simulink model "EvenOrOdd"  (R2021a)
settings: Solver=FixedStepDiscrete  StartTime=0.0  StopTime=10.0  RelTol=1e-3
settings Model: Creator=OmarMedhat  LastModifiedBy=OmarMedhat
settings OptimizationCC: DefaultParameterBehavior=Inlined  EnhancedBackFolding=on  PassReuseOutputArgsAs=Individual arguments  ZeroExternalMemoryAtStartup=off  ZeroInternalMemoryAtStartup=off  OptimizeBlockOrder=speed  DifferentSizesBufferReuse=on  OptimizationCustomize=off  EfficientTunableParamExpr=on
settings DebuggingCC: ParameterTunabilityLossMsg=error
settings SFSimCC: MATLABDynamicMemAlloc=off
settings RTWCC: SystemTargetFile=ert.tlc  GenCodeOnly=on  TemplateMakefile=ert_default_tmf  GenerateReport=on  IncludeHyperlinkInReport=on  LaunchReport=on  GenerateTraceInfo=on
settings CodeAppCC: ForceParamTrailComments=on  IgnoreCustomStorageClasses=off  OperatorAnnotations=on  SimulinkDataObjDesc=on  SFDataObjDesc=on  InsertBlockDesc=on
settings ERTTargetCC: TargetLangStandard=C99 (ISO)  GenerateSampleERTMain=on  InlinedParameterPlacement=NonHierarchical  ERTCustomFileTemplate=example_file_process.tlc

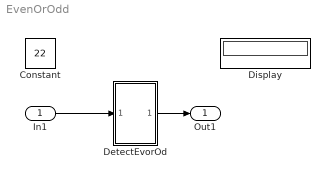
== system EvenOrOdd ==
  In1 : Inport
  Constant : Constant  Value=22
  DetectEvorOd : Subsystem  TreatAsAtomicUnit=on
      settings: RTWFcnNameOpts=Use subsystem name  RTWFileNameOpts=Use subsystem name
  Display : Display
  Out1 : Outport
  wires:
  In1/1 -> DetectEvorOd/1(In1)
  DetectEvorOd/1(Out1) -> Out1/1

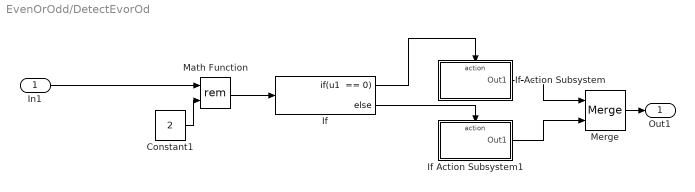
== system EvenOrOdd/DetectEvorOd ==
  In1 : Inport
  Constant1 : Constant  Value=2
  If : If  IfExpression="u1  == 0"
  If Action Subsystem : Subsystem  TreatAsAtomicUnit=on
  If Action Subsystem1 : Subsystem  TreatAsAtomicUnit=on
  Math Function : Math  Operator=rem  SaturateOnIntegerOverflow=on
  Merge : Merge
  Out1 : Outport
  wires:
  If/2 -> If Action Subsystem1/Action
  Constant1/1 -> Math Function/2
  Merge/1 -> Out1/1
  If Action Subsystem1/1(Out1) -> Merge/2
  If Action Subsystem/1(Out1) -> Merge/1
  If/1 -> If Action Subsystem/Action
  In1/1 -> Math Function/1
  Math Function/1 -> If/1

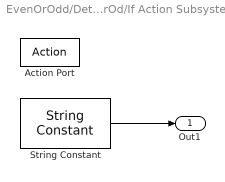
== system EvenOrOdd/DetectEvorOd/If Action Subsystem ==
  Action Port : ActionPort  ActionPortLabel="if(u1  == 0)"
  String Constant : StringConstant  String="\"Even\""
  Out1 : Outport
  wires:
  String Constant/1 -> Out1/1

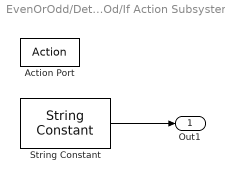
== system EvenOrOdd/DetectEvorOd/If Action Subsystem1 ==
  Action Port : ActionPort  ActionPortLabel=else
  String Constant : StringConstant  String="\"Odd\""
  Out1 : Outport
  wires:
  String Constant/1 -> Out1/1
